simulink model "gimbal_communication"  (R2017a)
settings: Solver=FixedStepAuto  StartTime=0.0  StopTime=1  FixedStep=0.02  RelTol=1e-3
undefined symbols (not defined in the file): serial
libraries: instrumentlib x3, aerolibanimutils x1
settings Model: SimulationMode=accelerator  Creator=s128701  LastModifiedBy=s128701
settings DataIOCC: ReturnWorkspaceOutputs=on

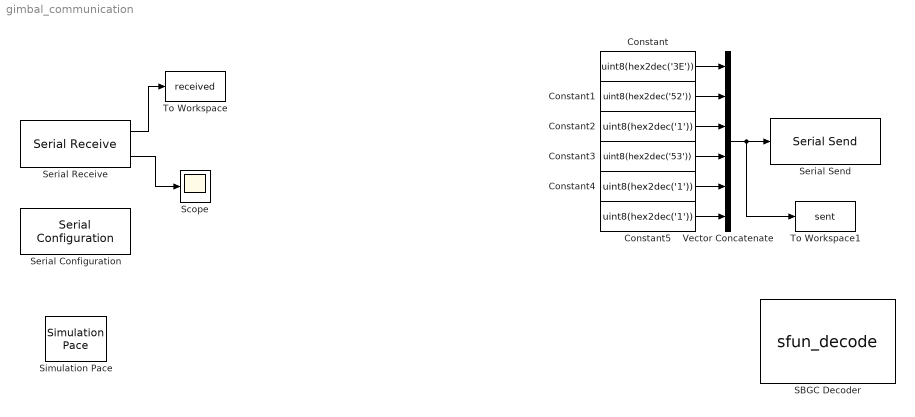
== system gimbal_communication ==
  Constant : Constant  Value=uint8(hex2dec('3E'))
  Constant1 : Constant  Value=uint8(hex2dec('52'))
  Constant2 : Constant  Value=uint8(hex2dec('1'))
  Constant3 : Constant  Value=uint8(hex2dec('53'))
  Constant4 : Constant  Value=uint8(hex2dec('1'))
  Constant5 : Constant  Value=uint8(hex2dec('1'))
  SBGC Decoder : S-Function  FunctionName=sfun_decode  SFunctionDeploymentMode=off  EnableBusSupport=off
  Scope : Scope
  Serial Configuration : instrumentlib/Serial Configuration  Priority=-200000  ComPortMenu=<Please select a port...>  ComPort=COM15  ObjConstructor=serial('COM15');  BaudRate=115200  DataBits=8  Parity=none  StopBits=1  FlowControl=none  Timeout=10  ByteOrder=LittleEndian
  Serial Receive : instrumentlib/Serial Receive  ComPortMenu=COM15  ComPort=COM15  ObjConstructor=serial('COM15');  Terminator=<none>  DataSize="[1  255]"  DataType=uint8  EnableBlockingMode=off  ActionDataUnavailable=Output custom value  CustomValue=zeros(1,255)  SampleTime=-1
  Serial Send : instrumentlib/Serial Send  ComPortMenu=COM15  ComPort=COM15  ObjConstructor=serial('COM15');  Terminator=<none>  EnableBlockingMode=on
  Simulation Pace : aerolibanimutils/Simulation Pace  SimulationPace=1  SleepMode=MATLAB Thread  OutputPaceError=off  SampleTime=-1
  To Workspace : ToWorkspace  VariableName=received  SaveFormat=Timeseries  SampleTime=-1
  To Workspace1 : ToWorkspace  VariableName=sent  SaveFormat=Timeseries  SampleTime=-1
  Vector Concatenate : Concatenate  NumInputs=6
  wires:
  Serial Receive/1 -> To Workspace/1
  Vector Concatenate/1 -> To Workspace1/1, Serial Send/1
  Constant/1 -> Vector Concatenate/1
  Constant1/1 -> Vector Concatenate/2
  Constant2/1 -> Vector Concatenate/3
  Constant3/1 -> Vector Concatenate/4
  Constant4/1 -> Vector Concatenate/5
  Constant5/1 -> Vector Concatenate/6
  Serial Receive/2 -> Scope/1
